simulink model "Podst"  (R2020b)
settings: Solver=ode23tb  StartTime=0.0  StopTime=0.2  MaxStep=10e-5  RelTol=1e-3
libraries: dspstat3 x40, powerlib x15, powerlib_meascontrol x5
settings Model: Creator=New-life  LastModifiedBy=New-life

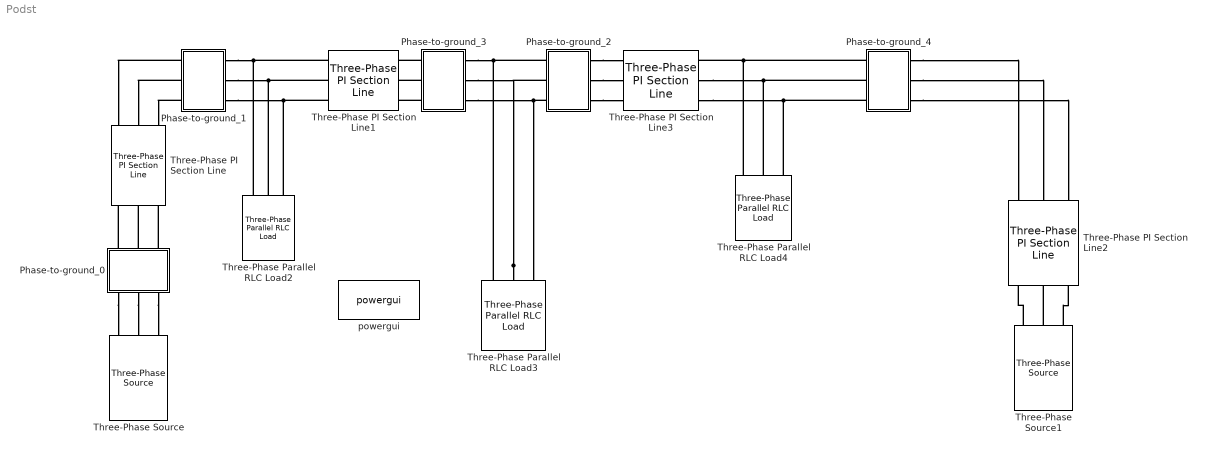
== system Podst ==
  Phase-to-ground_0 : Subsystem
      settings: CopyFcn=|
      | % Получаем путь и имя нового (только что скопированного) блока
      | blockPath = gcb;
      | blockName = get_param(blockPath, 'Name');
      | 
      | % Ищем число в названии самой подсистемы (например, берем "2" из "Measure_2")
      | numStr = regexp(blockName, '\d+', 'match');
      | 
      | if ~isempty(numStr)
      |     newNum = numStr{end}; % Берем последнее найденное число
      | 
      |     % --- 1. Обновляем скрытые теги в Goto и From (радиочастоты) ---
      |     gotos = find_system(blockPath, 'LookUnderMasks', 'on', 'BlockType', 'Goto');
      |     froms = find_system(blockPath, 'LookUnderMasks', 'on', 'BlockType', 'From');
      | 
      |     for i = 1:length(gotos)
      |         oldTag = get_param(gotos{i}, 'GotoTag');
      |         set_param(gotos{i}, 'GotoTag', regexprep(oldTag, '\d+$', newNum));
      |     end
      |     for i = 1:length(froms)
      |         oldTag = get_param(froms{i}, 'GotoTag');
      |         set_param(froms{i}, 'GotoTag', regexprep(oldTag, '\d+$', newNum));
      |     end
      | 
      |     % --- 2. ПЕРЕИМЕНОВЫВАЕМ САМИ БЛОКИ (визуальные надписи UI0 -> UI1 и т.д.) ---
      |     % Ищем все элементы только внутри этой подсистемы
      |     internalBlocks = find_system(blockPath, 'SearchDepth', 1, 'LookUnderMasks', 'on');
      | 
      |     % Цикл начинаем с 2, так как 1-й элемент в списке - это сама папка подсистемы
      |     for i = 2:length(internalBlocks)
      |         oldName = get_param(internalBlocks{i}, 'Name');
      |         % Ищем цифру в конце имени и меняем на новую
      |         newName = regexprep(oldName, '\d+$', newNum);
      | 
      |         % Если имя изменилось, применяем его
      |         if ~strcmp(oldName, newName)
      |             try
      |                 set_param(internalBlocks{i}, 'Name', newName);
      |             catch
      |                 % Игнорируем ошибку, если вдруг такое имя уже случайно есть
      |             end
      |         end
      |     end
      | end
  Phase-to-ground_1 : Subsystem
      settings: CopyFcn=|
      | % Получаем путь и имя нового (только что скопированного) блока
      | blockPath = gcb;
      | blockName = get_param(blockPath, 'Name');
      | 
      | % Ищем число в названии самой подсистемы (например, берем "2" из "Measure_2")
      | numStr = regexp(blockName, '\d+', 'match');
      | 
      | if ~isempty(numStr)
      |     newNum = numStr{end}; % Берем последнее найденное число
      | 
      |     % --- 1. Обновляем скрытые теги в Goto и From (радиочастоты) ---
      |     gotos = find_system(blockPath, 'LookUnderMasks', 'on', 'BlockType', 'Goto');
      |     froms = find_system(blockPath, 'LookUnderMasks', 'on', 'BlockType', 'From');
      | 
      |     for i = 1:length(gotos)
      |         oldTag = get_param(gotos{i}, 'GotoTag');
      |         set_param(gotos{i}, 'GotoTag', regexprep(oldTag, '\d+$', newNum));
      |     end
      |     for i = 1:length(froms)
      |         oldTag = get_param(froms{i}, 'GotoTag');
      |         set_param(froms{i}, 'GotoTag', regexprep(oldTag, '\d+$', newNum));
      |     end
      | 
      |     % --- 2. ПЕРЕИМЕНОВЫВАЕМ САМИ БЛОКИ (визуальные надписи UI0 -> UI1 и т.д.) ---
      |     % Ищем все элементы только внутри этой подсистемы
      |     internalBlocks = find_system(blockPath, 'SearchDepth', 1, 'LookUnderMasks', 'on');
      | 
      |     % Цикл начинаем с 2, так как 1-й элемент в списке - это сама папка подсистемы
      |     for i = 2:length(internalBlocks)
      |         oldName = get_param(internalBlocks{i}, 'Name');
      |         % Ищем цифру в конце имени и меняем на новую
      |         newName = regexprep(oldName, '\d+$', newNum);
      | 
      |         % Если имя изменилось, применяем его
      |         if ~strcmp(oldName, newName)
      |             try
      |                 set_param(internalBlocks{i}, 'Name', newName);
      |             catch
      |                 % Игнорируем ошибку, если вдруг такое имя уже случайно есть
      |             end
      |         end
      |     end
      | end
  Phase-to-ground_2 : Subsystem
      settings: CopyFcn=|
      | % Получаем путь и имя нового (только что скопированного) блока
      | blockPath = gcb;
      | blockName = get_param(blockPath, 'Name');
      | 
      | % Ищем число в названии самой подсистемы (например, берем "2" из "Measure_2")
      | numStr = regexp(blockName, '\d+', 'match');
      | 
      | if ~isempty(numStr)
      |     newNum = numStr{end}; % Берем последнее найденное число
      | 
      |     % --- 1. Обновляем скрытые теги в Goto и From (радиочастоты) ---
      |     gotos = find_system(blockPath, 'LookUnderMasks', 'on', 'BlockType', 'Goto');
      |     froms = find_system(blockPath, 'LookUnderMasks', 'on', 'BlockType', 'From');
      | 
      |     for i = 1:length(gotos)
      |         oldTag = get_param(gotos{i}, 'GotoTag');
      |         set_param(gotos{i}, 'GotoTag', regexprep(oldTag, '\d+$', newNum));
      |     end
      |     for i = 1:length(froms)
      |         oldTag = get_param(froms{i}, 'GotoTag');
      |         set_param(froms{i}, 'GotoTag', regexprep(oldTag, '\d+$', newNum));
      |     end
      | 
      |     % --- 2. ПЕРЕИМЕНОВЫВАЕМ САМИ БЛОКИ (визуальные надписи UI0 -> UI1 и т.д.) ---
      |     % Ищем все элементы только внутри этой подсистемы
      |     internalBlocks = find_system(blockPath, 'SearchDepth', 1, 'LookUnderMasks', 'on');
      | 
      |     % Цикл начинаем с 2, так как 1-й элемент в списке - это сама папка подсистемы
      |     for i = 2:length(internalBlocks)
      |         oldName = get_param(internalBlocks{i}, 'Name');
      |         % Ищем цифру в конце имени и меняем на новую
      |         newName = regexprep(oldName, '\d+$', newNum);
      | 
      |         % Если имя изменилось, применяем его
      |         if ~strcmp(oldName, newName)
      |             try
      |                 set_param(internalBlocks{i}, 'Name', newName);
      |             catch
      |                 % Игнорируем ошибку, если вдруг такое имя уже случайно есть
      |             end
      |         end
      |     end
      | end
  Phase-to-ground_3 : Subsystem
      settings: CopyFcn=|
      | % Получаем путь и имя нового (только что скопированного) блока
      | blockPath = gcb;
      | blockName = get_param(blockPath, 'Name');
      | 
      | % Ищем число в названии самой подсистемы (например, берем "2" из "Measure_2")
      | numStr = regexp(blockName, '\d+', 'match');
      | 
      | if ~isempty(numStr)
      |     newNum = numStr{end}; % Берем последнее найденное число
      | 
      |     % --- 1. Обновляем скрытые теги в Goto и From (радиочастоты) ---
      |     gotos = find_system(blockPath, 'LookUnderMasks', 'on', 'BlockType', 'Goto');
      |     froms = find_system(blockPath, 'LookUnderMasks', 'on', 'BlockType', 'From');
      | 
      |     for i = 1:length(gotos)
      |         oldTag = get_param(gotos{i}, 'GotoTag');
      |         set_param(gotos{i}, 'GotoTag', regexprep(oldTag, '\d+$', newNum));
      |     end
      |     for i = 1:length(froms)
      |         oldTag = get_param(froms{i}, 'GotoTag');
      |         set_param(froms{i}, 'GotoTag', regexprep(oldTag, '\d+$', newNum));
      |     end
      | 
      |     % --- 2. ПЕРЕИМЕНОВЫВАЕМ САМИ БЛОКИ (визуальные надписи UI0 -> UI1 и т.д.) ---
      |     % Ищем все элементы только внутри этой подсистемы
      |     internalBlocks = find_system(blockPath, 'SearchDepth', 1, 'LookUnderMasks', 'on');
      | 
      |     % Цикл начинаем с 2, так как 1-й элемент в списке - это сама папка подсистемы
      |     for i = 2:length(internalBlocks)
      |         oldName = get_param(internalBlocks{i}, 'Name');
      |         % Ищем цифру в конце имени и меняем на новую
      |         newName = regexprep(oldName, '\d+$', newNum);
      | 
      |         % Если имя изменилось, применяем его
      |         if ~strcmp(oldName, newName)
      |             try
      |                 set_param(internalBlocks{i}, 'Name', newName);
      |             catch
      |                 % Игнорируем ошибку, если вдруг такое имя уже случайно есть
      |             end
      |         end
      |     end
      | end
  Phase-to-ground_4 : Subsystem
      settings: CopyFcn=|
      | % Получаем путь и имя нового (только что скопированного) блока
      | blockPath = gcb;
      | blockName = get_param(blockPath, 'Name');
      | 
      | % Ищем число в названии самой подсистемы (например, берем "2" из "Measure_2")
      | numStr = regexp(blockName, '\d+', 'match');
      | 
      | if ~isempty(numStr)
      |     newNum = numStr{end}; % Берем последнее найденное число
      | 
      |     % --- 1. Обновляем скрытые теги в Goto и From (радиочастоты) ---
      |     gotos = find_system(blockPath, 'LookUnderMasks', 'on', 'BlockType', 'Goto');
      |     froms = find_system(blockPath, 'LookUnderMasks', 'on', 'BlockType', 'From');
      | 
      |     for i = 1:length(gotos)
      |         oldTag = get_param(gotos{i}, 'GotoTag');
      |         set_param(gotos{i}, 'GotoTag', regexprep(oldTag, '\d+$', newNum));
      |     end
      |     for i = 1:length(froms)
      |         oldTag = get_param(froms{i}, 'GotoTag');
      |         set_param(froms{i}, 'GotoTag', regexprep(oldTag, '\d+$', newNum));
      |     end
      | 
      |     % --- 2. ПЕРЕИМЕНОВЫВАЕМ САМИ БЛОКИ (визуальные надписи UI0 -> UI1 и т.д.) ---
      |     % Ищем все элементы только внутри этой подсистемы
      |     internalBlocks = find_system(blockPath, 'SearchDepth', 1, 'LookUnderMasks', 'on');
      | 
      |     % Цикл начинаем с 2, так как 1-й элемент в списке - это сама папка подсистемы
      |     for i = 2:length(internalBlocks)
      |         oldName = get_param(internalBlocks{i}, 'Name');
      |         % Ищем цифру в конце имени и меняем на новую
      |         newName = regexprep(oldName, '\d+$', newNum);
      | 
      |         % Если имя изменилось, применяем его
      |         if ~strcmp(oldName, newName)
      |             try
      |                 set_param(internalBlocks{i}, 'Name', newName);
      |             catch
      |                 % Игнорируем ошибку, если вдруг такое имя уже случайно есть
      |             end
      |         end
      |     end
      | end
  Three-Phase PI Section Line{,1..3} (4 alike) : powerlib/Elements/Three-Phase PI Section Line  LConnTagsString=a|b|c  RConnTagsString=A|B|C  Length=2  Frequency=50  Resistances=[ 0.42 0.3864]  Inductances="[ 1.248e-3  4.1264e-3]"  Capacitances=[1e-8 1e-8]
  Three-Phase Parallel RLC Load2 : powerlib/Elements/Three-Phase Parallel RLC Load  LConnTagsString=A|B|C  Configuration=Y (grounded)  NominalVoltage=10000  Vabc=[1e3 1e3 1e3]  Vabcp=[1e3 1e3 1e3]  NominalFrequency=50  UnbalancedPower=off  ActivePower=400e3  InductivePower=248e3  CapacitivePower=0  Pabc=[10e3 9e3 11e3]  QLabc=[100 90 110]  QCabc=[100 90 110]  Pabcp=[10e3 9e3 11e3]  QLabcp=[100 90 110]  QCabcp=[100 90 110]  Measurements=None  LoadType=constant Z
  Three-Phase Parallel RLC Load3 : powerlib/Elements/Three-Phase Parallel RLC Load  LConnTagsString=A|B|C  Configuration=Y (grounded)  NominalVoltage=10000  Vabc=[1e3 1e3 1e3]  Vabcp=[1e3 1e3 1e3]  NominalFrequency=50  UnbalancedPower=off  ActivePower=250e3  InductivePower=155e3  CapacitivePower=0  Pabc=[10e3 9e3 11e3]  QLabc=[100 90 110]  QCabc=[100 90 110]  Pabcp=[10e3 9e3 11e3]  QLabcp=[100 90 110]  QCabcp=[100 90 110]  Measurements=None  LoadType=constant Z
  Three-Phase Parallel RLC Load4 : powerlib/Elements/Three-Phase Parallel RLC Load  LConnTagsString=A|B|C  Configuration=Y (grounded)  NominalVoltage=10000  Vabc=[1e3 1e3 1e3]  Vabcp=[1e3 1e3 1e3]  NominalFrequency=50  UnbalancedPower=off  ActivePower=500e3  InductivePower=310e3  CapacitivePower=0  Pabc=[10e3 9e3 11e3]  QLabc=[100 90 110]  QCabc=[100 90 110]  Pabcp=[10e3 9e3 11e3]  QLabcp=[100 90 110]  QCabcp=[100 90 110]  Measurements=None  LoadType=constant Z
  Three-Phase Source : powerlib/Electrical Sources/Three-Phase Source  InternalConnection=Y  VoltagePhases=off  Voltage=10117  PhaseAngle=0  Voltage_phases=[25e3 25e3 25e3]/sqrt(3)  PhaseAngles_phases=[0 -120 +120]  Frequency=50  NonIdealSource=on  SpecifyImpedance=on  Resistance=0.8929  Inductance=16.58e-3  ShortCircuitLevel=100e10  BaseVoltage=25e3  XRratio=7  BusType=swing  Pref=10e3  Qref=0  Prefabc=[10e3, 10e3, 10e3]  Qrefabc=[0, 0, 0]  Qmin=-inf  Qmax=inf
  Three-Phase Source1 : powerlib/Electrical Sources/Three-Phase Source  InternalConnection=Y  VoltagePhases=off  Voltage=10117  PhaseAngle=0  Voltage_phases=[25e3 25e3 25e3]/sqrt(3)  PhaseAngles_phases=[0 -120 +120]  Frequency=50  NonIdealSource=on  SpecifyImpedance=on  Resistance=0.8929  Inductance=16.58e-3  ShortCircuitLevel=100e10  BaseVoltage=25e3  XRratio=7  BusType=swing  Pref=10e3  Qref=0  Prefabc=[10e3, 10e3, 10e3]  Qrefabc=[0, 0, 0]  Qmin=-inf  Qmax=inf
  powergui : powerlib/powergui  Priority=1  SimulationMode=Continuous  SampleTime=50e-6  frequency=60  Iterations=50  frequencyindice=50  Pbase=100e6  ErrMax=1e-4  UnitsV=kV  UnitsW=MW  buscounter=0  FunctionMessages=off  echomessages=off  EnableUseOfTLC=off  CurrentSourceSwitches=off  DisableSnubberDevices=off  DisableRonSwitches=off  DisableVfSwitches=off  DisplayEquations=off  AutomaticDiscreteSolvers=off  SolverType=Tustin/Backward Euler (TBE)  Interpol=off  ExternalGateDelay=off  methode=off  Ts=100  x0status=blocks  SPID=on  SwTol=0  HookPort=off  NonlinearTolerance=1e-4  nMaxIteration=100  ContinueOnMaxIteration=off  RestoreLinks=warning  ResistiveCurrentMeasurement=off  Frange=[0:2:500]  Ylog=off  Xlog=on  ShowGrid=off  save=off  variable=ZData  structure=0  ZoomFFT=off  StartTime=0.0  cycles=1  DisplayStyle=1  fundamental=60  FreqAxis=off  MaxFrequency=1000  frequencyindicesteady=1  RmsSteady=1  display=off
  connections:
  Phase-to-ground_0/LConn1 -- Three-Phase Source/RConn1
  Phase-to-ground_0/LConn2 -- Three-Phase Source/RConn2
  Three-Phase PI Section Line1/LConn1 -- Phase-to-ground_1/RConn1 -- Three-Phase Parallel RLC Load2/LConn1
  Three-Phase PI Section Line1/LConn2 -- Phase-to-ground_1/RConn2 -- Three-Phase Parallel RLC Load2/LConn2
  Three-Phase PI Section Line1/LConn3 -- Phase-to-ground_1/RConn3 -- Three-Phase Parallel RLC Load2/LConn3
  Three-Phase Source1/RConn2 -- Three-Phase PI Section Line2/RConn2
  Three-Phase Source1/RConn3 -- Three-Phase PI Section Line2/RConn3
  Three-Phase Source1/RConn1 -- Three-Phase PI Section Line2/RConn1
  Phase-to-ground_1/LConn1 -- Three-Phase PI Section Line/RConn1
  Phase-to-ground_1/LConn3 -- Three-Phase PI Section Line/RConn3
  Three-Phase Parallel RLC Load4/LConn1 -- Phase-to-ground_4/RConn1 -- Three-Phase PI Section Line3/RConn1
  Phase-to-ground_0/LConn3 -- Three-Phase Source/RConn3
  Phase-to-ground_0/RConn1 -- Three-Phase PI Section Line/LConn1
  Phase-to-ground_0/RConn2 -- Three-Phase PI Section Line/LConn2
  Phase-to-ground_0/RConn3 -- Three-Phase PI Section Line/LConn3
  Phase-to-ground_1/LConn2 -- Three-Phase PI Section Line/RConn2
  Phase-to-ground_2/LConn1 -- Three-Phase PI Section Line3/LConn1
  Phase-to-ground_3/LConn2 -- Three-Phase PI Section Line1/RConn2
  Phase-to-ground_3/RConn3 -- Phase-to-ground_2/RConn3 -- Three-Phase Parallel RLC Load3/LConn3
  Phase-to-ground_4/LConn1 -- Three-Phase PI Section Line2/LConn1
  Phase-to-ground_4/LConn2 -- Three-Phase PI Section Line2/LConn2
  Phase-to-ground_4/LConn3 -- Three-Phase PI Section Line2/LConn3
  Three-Phase PI Section Line3/RConn2 -- Phase-to-ground_4/RConn2 -- Three-Phase Parallel RLC Load4/LConn2
  Three-Phase PI Section Line3/RConn3 -- Phase-to-ground_4/RConn3 -- Three-Phase Parallel RLC Load4/LConn3
  Phase-to-ground_3/LConn1 -- Three-Phase PI Section Line1/RConn1
  Three-Phase Parallel RLC Load3/LConn2 -- Phase-to-ground_2/RConn2 -- Phase-to-ground_3/RConn2
  Phase-to-ground_3/LConn3 -- Three-Phase PI Section Line1/RConn3
  Phase-to-ground_2/LConn2 -- Three-Phase PI Section Line3/LConn2
  Phase-to-ground_3/RConn1 -- Three-Phase Parallel RLC Load3/LConn1 -- Phase-to-ground_2/RConn1
  Phase-to-ground_2/LConn3 -- Three-Phase PI Section Line3/LConn3

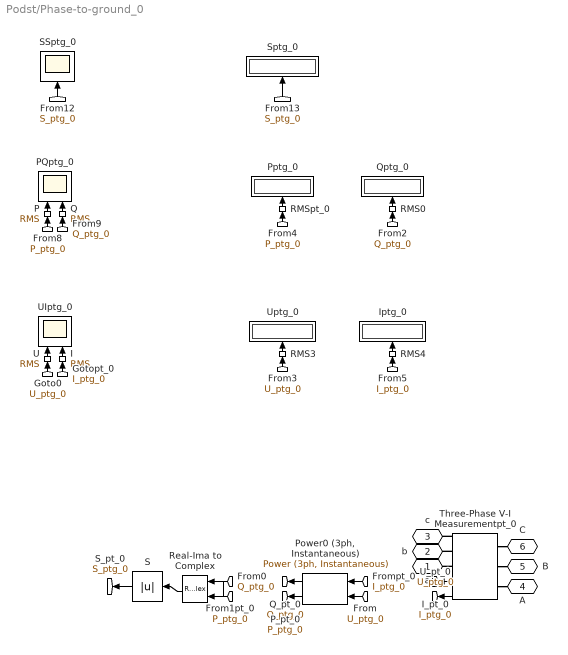
== system Podst/Phase-to-ground_0 ==
  I : dspstat3/RMS  run=off  directionMode=Each column  dimension=1  InputProcessing=Columns as channels (frame based)  reset_popup=None
  Iptg_0 : Display
      settings: Format=bank
  P : dspstat3/RMS  run=off  directionMode=Each column  dimension=1  InputProcessing=Columns as channels (frame based)  reset_popup=None
  PQptg_0 : Scope  NumInputPorts=2
  "Power0 (3ph, Instantaneous)" : powerlib_meascontrol/Measurements/Power (3ph, Instantaneous)
  Pptg_0 : Display
      settings: Format=bank
  Q : dspstat3/RMS  run=off  directionMode=Each column  dimension=1  InputProcessing=Columns as channels (frame based)  reset_popup=None
  Qptg_0 : Display
      settings: Format=bank
  RMS0 : dspstat3/RMS  run=off  directionMode=Each column  dimension=1  InputProcessing=Columns as channels (frame based)  reset_popup=None
  RMS3 : dspstat3/RMS  run=off  directionMode=Each column  dimension=1  InputProcessing=Columns as channels (frame based)  reset_popup=None
  RMS4 : dspstat3/RMS  run=off  directionMode=Each column  dimension=1  InputProcessing=Columns as channels (frame based)  reset_popup=None
  RMSpt_0 : dspstat3/RMS  run=off  directionMode=Each column  dimension=1  InputProcessing=Columns as channels (frame based)  reset_popup=None
  Real-Ima to Complex : RealImagToComplex
  S : Abs
  SSptg_0 : Scope
  Sptg_0 : Display
      settings: Format=bank
  Three-Phase V-I Measurementpt_0 : powerlib/Measurements/Three-Phase V-I Measurement  VoltageMeasurement=phase-to-ground  SetLabelV=off  LabelV=Vabc  Vpu=off  VpuLL=off  CurrentMeasurement=yes  SetLabelI=off  LabelI=Iabc  Ipu=off  Pbase=100e6  Vbase=500e3  OutputType=Complex  PhasorSimulation=off  PSBequivalent=0
  U : dspstat3/RMS  run=off  directionMode=Each column  dimension=1  InputProcessing=Columns as channels (frame based)  reset_popup=None
  UIptg_0 : Scope  NumInputPorts=2
  Uptg_0 : Display
      settings: Format=bank
  a : PMIOPort  Side=Right
  b : PMIOPort  Port=2  Side=Right
  c : PMIOPort  Port=3  Side=Right
  A : PMIOPort  Port=4  Side=Left
  B : PMIOPort  Port=5  Side=Left
  C : PMIOPort  Port=6  Side=Left
  tag scope: I_ptg_0=global, P_ptg_0=global, Q_ptg_0=global, S_ptg_0=global, U_ptg_0=global
  wires:
  S/1 -> [S_ptg_0]
  Real-Ima to Complex/1 -> S/1
  [P_ptg_0] -> P/1
  [S_ptg_0] -> Sptg_0/1
  [S_ptg_0] -> SSptg_0/1
  [P_ptg_0] -> RMSpt_0/1
  RMSpt_0/1 -> Pptg_0/1
  RMS0/1 -> Qptg_0/1
  [U_ptg_0] -> RMS3/1
  RMS3/1 -> Uptg_0/1
  [P_ptg_0] -> Real-Ima to Complex/1
  [Q_ptg_0] -> RMS0/1
  [I_ptg_0] -> RMS4/1
  RMS4/1 -> Iptg_0/1
  [U_ptg_0] -> U/1
  P/1 -> PQptg_0/1
  U/1 -> UIptg_0/1
  [I_ptg_0] -> I/1
  Three-Phase V-I Measurementpt_0/1 -> [U_ptg_0]
  [Q_ptg_0] -> Real-Ima to Complex/2
  Three-Phase V-I Measurementpt_0/2 -> [I_ptg_0]
  [Q_ptg_0] -> Q/1
  [U_ptg_0] -> "Power0 (3ph, Instantaneous)"/1
  [I_ptg_0] -> "Power0 (3ph, Instantaneous)"/2
  "Power0 (3ph, Instantaneous)"/2 -> [Q_ptg_0]
  "Power0 (3ph, Instantaneous)"/1 -> [P_ptg_0]
  I/1 -> UIptg_0/2
  Q/1 -> PQptg_0/2
  connections:
  Three-Phase V-I Measurementpt_0/LConn1 -- A/RConn1
  Three-Phase V-I Measurementpt_0/RConn1 -- a/RConn1
  Three-Phase V-I Measurementpt_0/LConn2 -- B/RConn1
  Three-Phase V-I Measurementpt_0/LConn3 -- C/RConn1
  Three-Phase V-I Measurementpt_0/RConn3 -- c/RConn1
  Three-Phase V-I Measurementpt_0/RConn2 -- b/RConn1

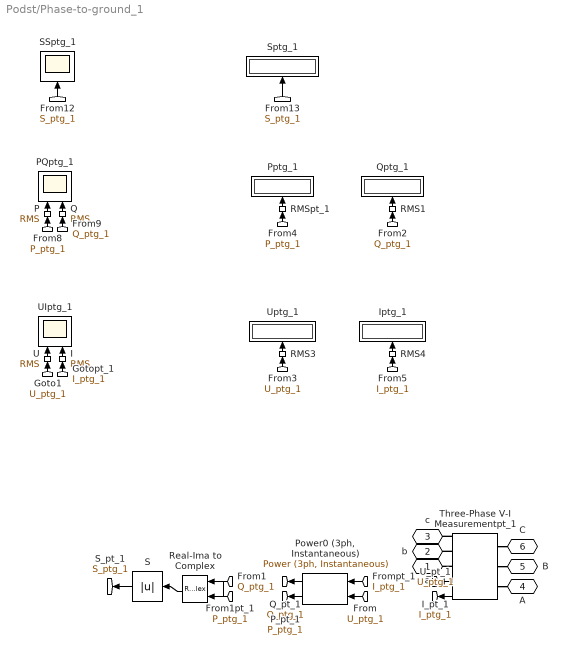
== system Podst/Phase-to-ground_1 ==
  I : dspstat3/RMS  run=off  directionMode=Each column  dimension=1  InputProcessing=Columns as channels (frame based)  reset_popup=None
  Iptg_1 : Display
      settings: Format=bank
  P : dspstat3/RMS  run=off  directionMode=Each column  dimension=1  InputProcessing=Columns as channels (frame based)  reset_popup=None
  PQptg_1 : Scope  NumInputPorts=2
  "Power0 (3ph, Instantaneous)" : powerlib_meascontrol/Measurements/Power (3ph, Instantaneous)
  Pptg_1 : Display
      settings: Format=bank
  Q : dspstat3/RMS  run=off  directionMode=Each column  dimension=1  InputProcessing=Columns as channels (frame based)  reset_popup=None
  Qptg_1 : Display
      settings: Format=bank
  RMS1 : dspstat3/RMS  run=off  directionMode=Each column  dimension=1  InputProcessing=Columns as channels (frame based)  reset_popup=None
  RMS3 : dspstat3/RMS  run=off  directionMode=Each column  dimension=1  InputProcessing=Columns as channels (frame based)  reset_popup=None
  RMS4 : dspstat3/RMS  run=off  directionMode=Each column  dimension=1  InputProcessing=Columns as channels (frame based)  reset_popup=None
  RMSpt_1 : dspstat3/RMS  run=off  directionMode=Each column  dimension=1  InputProcessing=Columns as channels (frame based)  reset_popup=None
  Real-Ima to Complex : RealImagToComplex
  S : Abs
  SSptg_1 : Scope
  Sptg_1 : Display
      settings: Format=bank
  Three-Phase V-I Measurementpt_1 : powerlib/Measurements/Three-Phase V-I Measurement  VoltageMeasurement=phase-to-ground  SetLabelV=off  LabelV=Vabc  Vpu=off  VpuLL=off  CurrentMeasurement=yes  SetLabelI=off  LabelI=Iabc  Ipu=off  Pbase=100e6  Vbase=500e3  OutputType=Complex  PhasorSimulation=off  PSBequivalent=0
  U : dspstat3/RMS  run=off  directionMode=Each column  dimension=1  InputProcessing=Columns as channels (frame based)  reset_popup=None
  UIptg_1 : Scope  NumInputPorts=2
  Uptg_1 : Display
      settings: Format=bank
  a : PMIOPort  Side=Right
  b : PMIOPort  Port=2  Side=Right
  c : PMIOPort  Port=3  Side=Right
  A : PMIOPort  Port=4  Side=Left
  B : PMIOPort  Port=5  Side=Left
  C : PMIOPort  Port=6  Side=Left
  tag scope: I_ptg_1=global, P_ptg_1=global, Q_ptg_1=global, S_ptg_1=global, U_ptg_1=global
  wires:
  Q/1 -> PQptg_1/2
  I/1 -> UIptg_1/2
  "Power0 (3ph, Instantaneous)"/1 -> [P_ptg_1]
  "Power0 (3ph, Instantaneous)"/2 -> [Q_ptg_1]
  [I_ptg_1] -> "Power0 (3ph, Instantaneous)"/2
  [U_ptg_1] -> "Power0 (3ph, Instantaneous)"/1
  [Q_ptg_1] -> Q/1
  Three-Phase V-I Measurementpt_1/2 -> [I_ptg_1]
  [Q_ptg_1] -> Real-Ima to Complex/2
  Three-Phase V-I Measurementpt_1/1 -> [U_ptg_1]
  [I_ptg_1] -> I/1
  U/1 -> UIptg_1/1
  P/1 -> PQptg_1/1
  [U_ptg_1] -> U/1
  RMS4/1 -> Iptg_1/1
  [I_ptg_1] -> RMS4/1
  [Q_ptg_1] -> RMS1/1
  [P_ptg_1] -> Real-Ima to Complex/1
  RMS3/1 -> Uptg_1/1
  [U_ptg_1] -> RMS3/1
  RMS1/1 -> Qptg_1/1
  RMSpt_1/1 -> Pptg_1/1
  [P_ptg_1] -> RMSpt_1/1
  [S_ptg_1] -> SSptg_1/1
  [S_ptg_1] -> Sptg_1/1
  [P_ptg_1] -> P/1
  Real-Ima to Complex/1 -> S/1
  S/1 -> [S_ptg_1]
  connections:
  Three-Phase V-I Measurementpt_1/RConn2 -- b/RConn1
  Three-Phase V-I Measurementpt_1/RConn3 -- c/RConn1
  Three-Phase V-I Measurementpt_1/LConn3 -- C/RConn1
  Three-Phase V-I Measurementpt_1/LConn2 -- B/RConn1
  Three-Phase V-I Measurementpt_1/RConn1 -- a/RConn1
  Three-Phase V-I Measurementpt_1/LConn1 -- A/RConn1

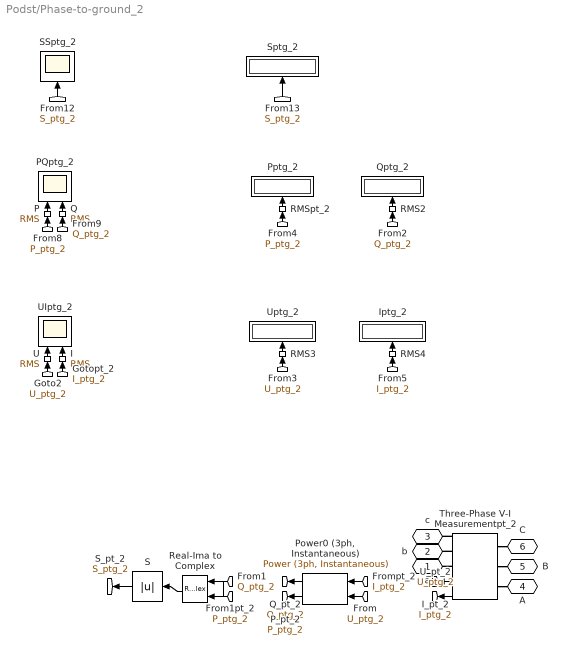
== system Podst/Phase-to-ground_2 ==
  I : dspstat3/RMS  run=off  directionMode=Each column  dimension=1  InputProcessing=Columns as channels (frame based)  reset_popup=None
  Iptg_2 : Display
      settings: Format=bank
  P : dspstat3/RMS  run=off  directionMode=Each column  dimension=1  InputProcessing=Columns as channels (frame based)  reset_popup=None
  PQptg_2 : Scope  NumInputPorts=2
  "Power0 (3ph, Instantaneous)" : powerlib_meascontrol/Measurements/Power (3ph, Instantaneous)
  Pptg_2 : Display
      settings: Format=bank
  Q : dspstat3/RMS  run=off  directionMode=Each column  dimension=1  InputProcessing=Columns as channels (frame based)  reset_popup=None
  Qptg_2 : Display
      settings: Format=bank
  RMS2 : dspstat3/RMS  run=off  directionMode=Each column  dimension=1  InputProcessing=Columns as channels (frame based)  reset_popup=None
  RMS3 : dspstat3/RMS  run=off  directionMode=Each column  dimension=1  InputProcessing=Columns as channels (frame based)  reset_popup=None
  RMS4 : dspstat3/RMS  run=off  directionMode=Each column  dimension=1  InputProcessing=Columns as channels (frame based)  reset_popup=None
  RMSpt_2 : dspstat3/RMS  run=off  directionMode=Each column  dimension=1  InputProcessing=Columns as channels (frame based)  reset_popup=None
  Real-Ima to Complex : RealImagToComplex
  S : Abs
  SSptg_2 : Scope
  Sptg_2 : Display
      settings: Format=bank
  Three-Phase V-I Measurementpt_2 : powerlib/Measurements/Three-Phase V-I Measurement  VoltageMeasurement=phase-to-ground  SetLabelV=off  LabelV=Vabc  Vpu=off  VpuLL=off  CurrentMeasurement=yes  SetLabelI=off  LabelI=Iabc  Ipu=off  Pbase=100e6  Vbase=500e3  OutputType=Complex  PhasorSimulation=off  PSBequivalent=0
  U : dspstat3/RMS  run=off  directionMode=Each column  dimension=1  InputProcessing=Columns as channels (frame based)  reset_popup=None
  UIptg_2 : Scope  NumInputPorts=2
  Uptg_2 : Display
      settings: Format=bank
  a : PMIOPort  Side=Right
  b : PMIOPort  Port=2  Side=Right
  c : PMIOPort  Port=3  Side=Right
  A : PMIOPort  Port=4  Side=Left
  B : PMIOPort  Port=5  Side=Left
  C : PMIOPort  Port=6  Side=Left
  tag scope: I_ptg_2=global, P_ptg_2=global, Q_ptg_2=global, S_ptg_2=global, U_ptg_2=global
  wires:
  S/1 -> [S_ptg_2]
  Real-Ima to Complex/1 -> S/1
  [P_ptg_2] -> P/1
  [S_ptg_2] -> Sptg_2/1
  [S_ptg_2] -> SSptg_2/1
  [P_ptg_2] -> RMSpt_2/1
  RMSpt_2/1 -> Pptg_2/1
  RMS2/1 -> Qptg_2/1
  [U_ptg_2] -> RMS3/1
  RMS3/1 -> Uptg_2/1
  [P_ptg_2] -> Real-Ima to Complex/1
  [Q_ptg_2] -> RMS2/1
  [I_ptg_2] -> RMS4/1
  RMS4/1 -> Iptg_2/1
  [U_ptg_2] -> U/1
  P/1 -> PQptg_2/1
  U/1 -> UIptg_2/1
  [I_ptg_2] -> I/1
  Three-Phase V-I Measurementpt_2/1 -> [U_ptg_2]
  [Q_ptg_2] -> Real-Ima to Complex/2
  Three-Phase V-I Measurementpt_2/2 -> [I_ptg_2]
  [Q_ptg_2] -> Q/1
  [U_ptg_2] -> "Power0 (3ph, Instantaneous)"/1
  [I_ptg_2] -> "Power0 (3ph, Instantaneous)"/2
  "Power0 (3ph, Instantaneous)"/2 -> [Q_ptg_2]
  "Power0 (3ph, Instantaneous)"/1 -> [P_ptg_2]
  I/1 -> UIptg_2/2
  Q/1 -> PQptg_2/2
  connections:
  Three-Phase V-I Measurementpt_2/LConn1 -- A/RConn1
  Three-Phase V-I Measurementpt_2/RConn1 -- a/RConn1
  Three-Phase V-I Measurementpt_2/LConn2 -- B/RConn1
  Three-Phase V-I Measurementpt_2/LConn3 -- C/RConn1
  Three-Phase V-I Measurementpt_2/RConn3 -- c/RConn1
  Three-Phase V-I Measurementpt_2/RConn2 -- b/RConn1

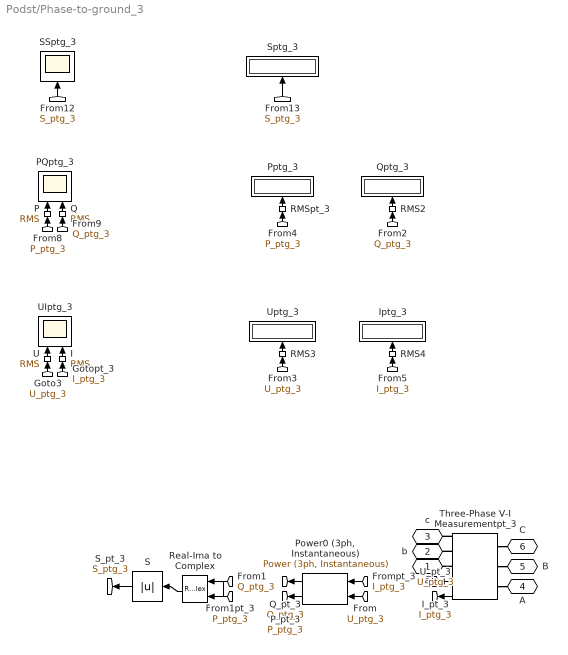
== system Podst/Phase-to-ground_3 ==
  I : dspstat3/RMS  run=off  directionMode=Each column  dimension=1  InputProcessing=Columns as channels (frame based)  reset_popup=None
  Iptg_3 : Display
      settings: Format=bank
  P : dspstat3/RMS  run=off  directionMode=Each column  dimension=1  InputProcessing=Columns as channels (frame based)  reset_popup=None
  PQptg_3 : Scope  NumInputPorts=2
  "Power0 (3ph, Instantaneous)" : powerlib_meascontrol/Measurements/Power (3ph, Instantaneous)
  Pptg_3 : Display
      settings: Format=bank
  Q : dspstat3/RMS  run=off  directionMode=Each column  dimension=1  InputProcessing=Columns as channels (frame based)  reset_popup=None
  Qptg_3 : Display
      settings: Format=bank
  RMS2 : dspstat3/RMS  run=off  directionMode=Each column  dimension=1  InputProcessing=Columns as channels (frame based)  reset_popup=None
  RMS3 : dspstat3/RMS  run=off  directionMode=Each column  dimension=1  InputProcessing=Columns as channels (frame based)  reset_popup=None
  RMS4 : dspstat3/RMS  run=off  directionMode=Each column  dimension=1  InputProcessing=Columns as channels (frame based)  reset_popup=None
  RMSpt_3 : dspstat3/RMS  run=off  directionMode=Each column  dimension=1  InputProcessing=Columns as channels (frame based)  reset_popup=None
  Real-Ima to Complex : RealImagToComplex
  S : Abs
  SSptg_3 : Scope
  Sptg_3 : Display
      settings: Format=bank
  Three-Phase V-I Measurementpt_3 : powerlib/Measurements/Three-Phase V-I Measurement  VoltageMeasurement=phase-to-ground  SetLabelV=off  LabelV=Vabc  Vpu=off  VpuLL=off  CurrentMeasurement=yes  SetLabelI=off  LabelI=Iabc  Ipu=off  Pbase=100e6  Vbase=500e3  OutputType=Complex  PhasorSimulation=off  PSBequivalent=0
  U : dspstat3/RMS  run=off  directionMode=Each column  dimension=1  InputProcessing=Columns as channels (frame based)  reset_popup=None
  UIptg_3 : Scope  NumInputPorts=2
  Uptg_3 : Display
      settings: Format=bank
  a : PMIOPort  Side=Right
  b : PMIOPort  Port=2  Side=Right
  c : PMIOPort  Port=3  Side=Right
  A : PMIOPort  Port=4  Side=Left
  B : PMIOPort  Port=5  Side=Left
  C : PMIOPort  Port=6  Side=Left
  tag scope: I_ptg_3=global, P_ptg_3=global, Q_ptg_3=global, S_ptg_3=global, U_ptg_3=global
  wires:
  Q/1 -> PQptg_3/2
  I/1 -> UIptg_3/2
  "Power0 (3ph, Instantaneous)"/1 -> [P_ptg_3]
  "Power0 (3ph, Instantaneous)"/2 -> [Q_ptg_3]
  [I_ptg_3] -> "Power0 (3ph, Instantaneous)"/2
  [U_ptg_3] -> "Power0 (3ph, Instantaneous)"/1
  [Q_ptg_3] -> Q/1
  Three-Phase V-I Measurementpt_3/2 -> [I_ptg_3]
  [Q_ptg_3] -> Real-Ima to Complex/2
  Three-Phase V-I Measurementpt_3/1 -> [U_ptg_3]
  [I_ptg_3] -> I/1
  U/1 -> UIptg_3/1
  P/1 -> PQptg_3/1
  [U_ptg_3] -> U/1
  RMS4/1 -> Iptg_3/1
  [I_ptg_3] -> RMS4/1
  [Q_ptg_3] -> RMS2/1
  [P_ptg_3] -> Real-Ima to Complex/1
  RMS3/1 -> Uptg_3/1
  [U_ptg_3] -> RMS3/1
  RMS2/1 -> Qptg_3/1
  RMSpt_3/1 -> Pptg_3/1
  [P_ptg_3] -> RMSpt_3/1
  [S_ptg_3] -> SSptg_3/1
  [S_ptg_3] -> Sptg_3/1
  [P_ptg_3] -> P/1
  Real-Ima to Complex/1 -> S/1
  S/1 -> [S_ptg_3]
  connections:
  Three-Phase V-I Measurementpt_3/RConn2 -- b/RConn1
  Three-Phase V-I Measurementpt_3/RConn3 -- c/RConn1
  Three-Phase V-I Measurementpt_3/LConn3 -- C/RConn1
  Three-Phase V-I Measurementpt_3/LConn2 -- B/RConn1
  Three-Phase V-I Measurementpt_3/RConn1 -- a/RConn1
  Three-Phase V-I Measurementpt_3/LConn1 -- A/RConn1

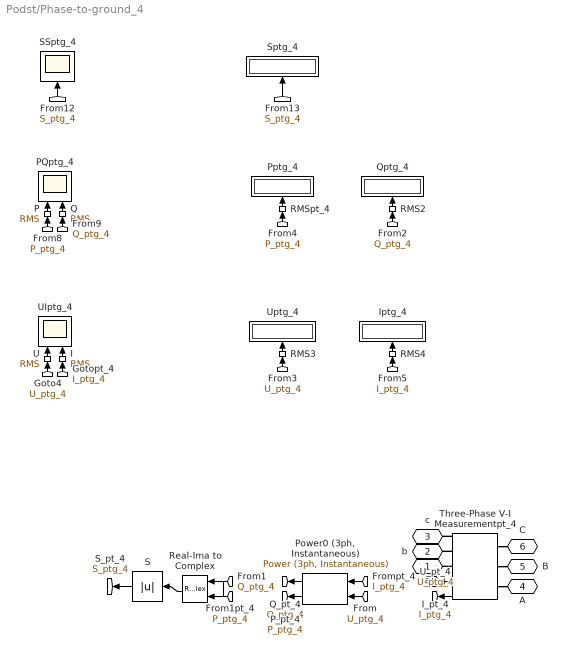
== system Podst/Phase-to-ground_4 ==
  I : dspstat3/RMS  run=off  directionMode=Each column  dimension=1  InputProcessing=Columns as channels (frame based)  reset_popup=None
  Iptg_4 : Display
      settings: Format=bank
  P : dspstat3/RMS  run=off  directionMode=Each column  dimension=1  InputProcessing=Columns as channels (frame based)  reset_popup=None
  PQptg_4 : Scope  NumInputPorts=2
  "Power0 (3ph, Instantaneous)" : powerlib_meascontrol/Measurements/Power (3ph, Instantaneous)
  Pptg_4 : Display
      settings: Format=bank
  Q : dspstat3/RMS  run=off  directionMode=Each column  dimension=1  InputProcessing=Columns as channels (frame based)  reset_popup=None
  Qptg_4 : Display
      settings: Format=bank
  RMS2 : dspstat3/RMS  run=off  directionMode=Each column  dimension=1  InputProcessing=Columns as channels (frame based)  reset_popup=None
  RMS3 : dspstat3/RMS  run=off  directionMode=Each column  dimension=1  InputProcessing=Columns as channels (frame based)  reset_popup=None
  RMS4 : dspstat3/RMS  run=off  directionMode=Each column  dimension=1  InputProcessing=Columns as channels (frame based)  reset_popup=None
  RMSpt_4 : dspstat3/RMS  run=off  directionMode=Each column  dimension=1  InputProcessing=Columns as channels (frame based)  reset_popup=None
  Real-Ima to Complex : RealImagToComplex
  S : Abs
  SSptg_4 : Scope
  Sptg_4 : Display
      settings: Format=bank
  Three-Phase V-I Measurementpt_4 : powerlib/Measurements/Three-Phase V-I Measurement  VoltageMeasurement=phase-to-ground  SetLabelV=off  LabelV=Vabc  Vpu=off  VpuLL=off  CurrentMeasurement=yes  SetLabelI=off  LabelI=Iabc  Ipu=off  Pbase=100e6  Vbase=500e3  OutputType=Complex  PhasorSimulation=off  PSBequivalent=0
  U : dspstat3/RMS  run=off  directionMode=Each column  dimension=1  InputProcessing=Columns as channels (frame based)  reset_popup=None
  UIptg_4 : Scope  NumInputPorts=2
  Uptg_4 : Display
      settings: Format=bank
  a : PMIOPort  Side=Right
  b : PMIOPort  Port=2  Side=Right
  c : PMIOPort  Port=3  Side=Right
  A : PMIOPort  Port=4  Side=Left
  B : PMIOPort  Port=5  Side=Left
  C : PMIOPort  Port=6  Side=Left
  tag scope: I_ptg_4=global, P_ptg_4=global, Q_ptg_4=global, S_ptg_4=global, U_ptg_4=global
  wires:
  Q/1 -> PQptg_4/2
  I/1 -> UIptg_4/2
  "Power0 (3ph, Instantaneous)"/1 -> [P_ptg_4]
  "Power0 (3ph, Instantaneous)"/2 -> [Q_ptg_4]
  [I_ptg_4] -> "Power0 (3ph, Instantaneous)"/2
  [U_ptg_4] -> "Power0 (3ph, Instantaneous)"/1
  [Q_ptg_4] -> Q/1
  Three-Phase V-I Measurementpt_4/2 -> [I_ptg_4]
  [Q_ptg_4] -> Real-Ima to Complex/2
  Three-Phase V-I Measurementpt_4/1 -> [U_ptg_4]
  [I_ptg_4] -> I/1
  U/1 -> UIptg_4/1
  P/1 -> PQptg_4/1
  [U_ptg_4] -> U/1
  RMS4/1 -> Iptg_4/1
  [I_ptg_4] -> RMS4/1
  [Q_ptg_4] -> RMS2/1
  [P_ptg_4] -> Real-Ima to Complex/1
  RMS3/1 -> Uptg_4/1
  [U_ptg_4] -> RMS3/1
  RMS2/1 -> Qptg_4/1
  RMSpt_4/1 -> Pptg_4/1
  [P_ptg_4] -> RMSpt_4/1
  [S_ptg_4] -> SSptg_4/1
  [S_ptg_4] -> Sptg_4/1
  [P_ptg_4] -> P/1
  Real-Ima to Complex/1 -> S/1
  S/1 -> [S_ptg_4]
  connections:
  Three-Phase V-I Measurementpt_4/RConn2 -- b/RConn1
  Three-Phase V-I Measurementpt_4/RConn3 -- c/RConn1
  Three-Phase V-I Measurementpt_4/LConn3 -- C/RConn1
  Three-Phase V-I Measurementpt_4/LConn2 -- B/RConn1
  Three-Phase V-I Measurementpt_4/RConn1 -- a/RConn1
  Three-Phase V-I Measurementpt_4/LConn1 -- A/RConn1
